simulink model "descriptor"  (R2015a)
settings: Solver=ode45  StartTime=0.0  StopTime=10.0  RelTol=1e-3
InitFcn:
  | %% DSPBuilder Start
  | alt_dspbuilder_update_model(bdroot)
  | %% DSPBuilder End
libraries: allblocks_alteradspbuilder2 x126
settings Model: Creator=ASUS  LastModifiedBy=ASUS

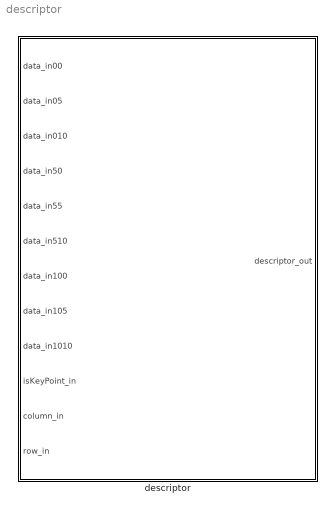
== system descriptor ==
  descriptor : Subsystem

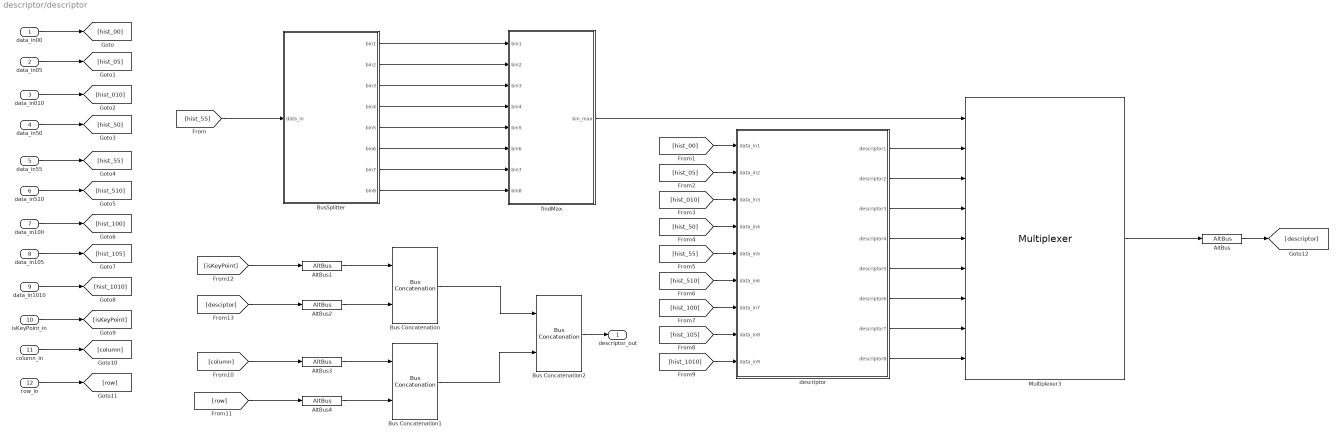
== system descriptor/descriptor ==
  data_in00 : Inport
  data_in05 : Inport  Port=2
  data_in010 : Inport  Port=3
  data_in50 : Inport  Port=4
  data_in55 : Inport  Port=5
  data_in510 : Inport  Port=6
  data_in100 : Inport  Port=7
  data_in105 : Inport  Port=8
  data_in1010 : Inport  Port=9
  isKeyPoint_in : Inport  Port=10
  column_in : Inport  Port=11
  row_in : Inport  Port=12
  AltBus : allblocks_alteradspbuilder2/AltBus  BusType=Unsigned Integer  bwl=128*9  bwr=0  saturate=off  floatingPointInput=on  floatingPointOutput=on  logOutputs=off  logFile=C:\Users\ASUS\Desktop\sift_fpga_final\Octave_1\tb_descriptor\descriptor_descriptor_AltBus.fixedpointlog
  AltBus1 : allblocks_alteradspbuilder2/AltBus  BusType=Single Bit  bwl=1  bwr=0  saturate=off  floatingPointInput=on  floatingPointOutput=on  logOutputs=off  logFile=C:\Users\ASUS\Desktop\sift_fpga_final\Octave_1\tb_descriptor\descriptor_descriptor_AltBus1.fixedpointlog
  AltBus2 : allblocks_alteradspbuilder2/AltBus  BusType=Unsigned Integer  bwl=128*9  bwr=0  saturate=off  floatingPointInput=on  floatingPointOutput=on  logOutputs=off  logFile=C:\Users\ASUS\Desktop\sift_fpga_final\Octave_1\tb_descriptor\descriptor_descriptor_AltBus2.fixedpointlog
  AltBus3 : allblocks_alteradspbuilder2/AltBus  BusType=Unsigned Integer  bwl=10  bwr=0  saturate=off  floatingPointInput=on  floatingPointOutput=on  logOutputs=off  logFile=C:\Users\ASUS\Desktop\sift_fpga_final\Octave_1\tb_descriptor\descriptor_descriptor_AltBus3.fixedpointlog
  AltBus4 : allblocks_alteradspbuilder2/AltBus  BusType=Unsigned Integer  bwl=10  bwr=0  saturate=off  floatingPointInput=on  floatingPointOutput=on  logOutputs=off  logFile=C:\Users\ASUS\Desktop\sift_fpga_final\Octave_1\tb_descriptor\descriptor_descriptor_AltBus4.fixedpointlog
  Bus Concatenation : allblocks_alteradspbuilder2/Bus Concatenation  isSigned=off  awidth=1  bwidth=128*9  pipeline_display=0
  Bus Concatenation1 : allblocks_alteradspbuilder2/Bus Concatenation  isSigned=off  awidth=10  bwidth=10  pipeline_display=0
  Bus Concatenation2 : allblocks_alteradspbuilder2/Bus Concatenation  isSigned=off  awidth=1153  bwidth=20  pipeline_display=0
  BusSplitter : Subsystem
  Multiplexer3 : allblocks_alteradspbuilder2/Multiplexer  numInputs=8  pipeline=0  oneHot=off  pipeline_display=0  use_ena=off  use_aclr=off  allowFloatingPointOverride=on  logOutputs=off  logFile=C:\Users\ASUS\Desktop\sift_fpga_final\Octave_1\tb_descriptor\descriptor_descriptor_Multiplexer3.fixedpointlog
  descriptor : Subsystem
  findMax : Subsystem
  descriptor_out : Outport
  wires:
  [hist_105] -> descriptor/8(data_in8)
  [hist_100] -> descriptor/7(data_in7)
  [hist_510] -> descriptor/6(data_in6)
  [hist_55] -> descriptor/5(data_in5)
  Multiplexer3/1 -> AltBus/1
  [hist_1010] -> descriptor/9(data_in9)
  descriptor/1(descriptor1) -> Multiplexer3/2
  [hist_05] -> descriptor/2(data_in2)
  [hist_010] -> descriptor/3(data_in3)
  [hist_50] -> descriptor/4(data_in4)
  descriptor/5(descriptor5) -> Multiplexer3/6
  descriptor/4(descriptor4) -> Multiplexer3/5
  [hist_00] -> descriptor/1(data_in1)
  descriptor/7(descriptor7) -> Multiplexer3/8
  descriptor/8(descriptor8) -> Multiplexer3/9
  descriptor/2(descriptor2) -> Multiplexer3/3
  descriptor/3(descriptor3) -> Multiplexer3/4
  descriptor/6(descriptor6) -> Multiplexer3/7
  BusSplitter/3(bin3) -> findMax/3(bin3)
  data_in00/1 -> [hist_00]
  data_in50/1 -> [hist_50]
  BusSplitter/1(bin1) -> findMax/1(bin1)
  data_in100/1 -> [hist_100]
  data_in010/1 -> [hist_010]
  data_in105/1 -> [hist_105]
  [hist_55] -> BusSplitter/1(data_in)
  data_in510/1 -> [hist_510]
  column_in/1 -> [column]
  data_in1010/1 -> [hist_1010]
  BusSplitter/8(bin8) -> findMax/8(bin8)
  findMax/1(bin_max) -> Multiplexer3/1
  data_in55/1 -> [hist_55]
  isKeyPoint_in/1 -> [isKeyPoint]
  row_in/1 -> [row]
  BusSplitter/4(bin4) -> findMax/4(bin4)
  BusSplitter/2(bin2) -> findMax/2(bin2)
  data_in05/1 -> [hist_05]
  BusSplitter/5(bin5) -> findMax/5(bin5)
  BusSplitter/7(bin7) -> findMax/7(bin7)
  BusSplitter/6(bin6) -> findMax/6(bin6)
  AltBus/1 -> [descriptor]
  [isKeyPoint] -> AltBus1/1
  [desciptor] -> AltBus2/1
  [column] -> AltBus3/1
  [row] -> AltBus4/1
  AltBus1/1 -> Bus Concatenation/1
  AltBus2/1 -> Bus Concatenation/2
  AltBus3/1 -> Bus Concatenation1/1
  AltBus4/1 -> Bus Concatenation1/2
  Bus Concatenation/1 -> Bus Concatenation2/1
  Bus Concatenation1/1 -> Bus Concatenation2/2
  Bus Concatenation2/1 -> descriptor_out/1

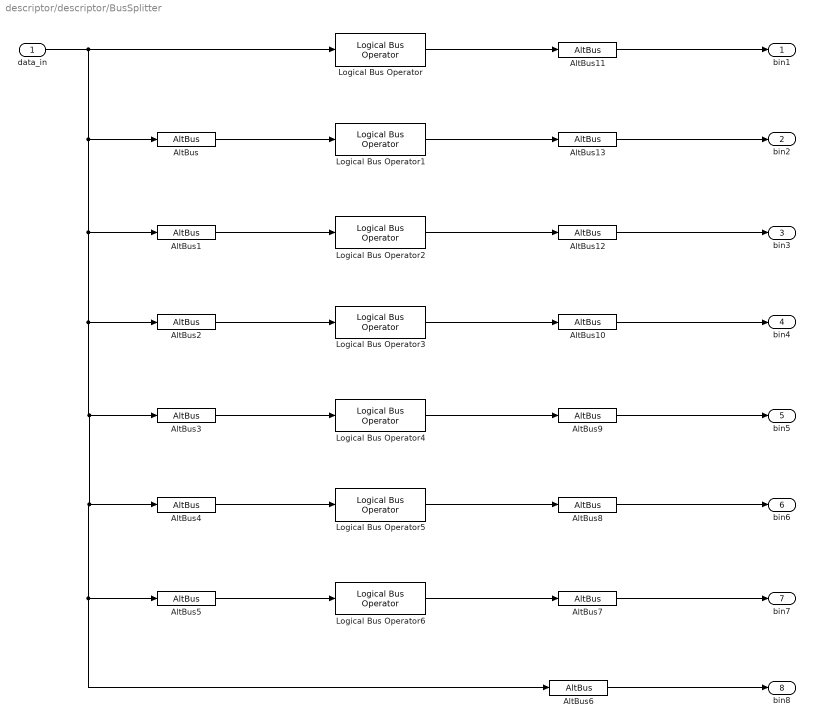
== system descriptor/descriptor/BusSplitter ==
  data_in : Inport
  AltBus : allblocks_alteradspbuilder2/AltBus  BusType=Unsigned Integer  bwl=112  bwr=0  saturate=off  floatingPointInput=on  floatingPointOutput=on  logOutputs=off  logFile=C:\Users\ASUS\Desktop\sift_fpga_final\Octave_1\tb_descriptor\descriptor_descriptor_BusSplitter_AltBus.fixedpointlog
  AltBus1 : allblocks_alteradspbuilder2/AltBus  BusType=Unsigned Integer  bwl=96  bwr=0  saturate=off  floatingPointInput=on  floatingPointOutput=on  logOutputs=off  logFile=C:\Users\ASUS\Desktop\sift_fpga_final\Octave_1\tb_descriptor\descriptor_descriptor_BusSplitter_AltBus1.fixedpointlog
  AltBus10 : allblocks_alteradspbuilder2/AltBus  BusType=Unsigned Integer  bwl=16  bwr=0  saturate=off  floatingPointInput=on  floatingPointOutput=on  logOutputs=off  logFile=C:\Users\ASUS\Desktop\sift_fpga_final\Octave_1\tb_descriptor\descriptor_descriptor_BusSplitter_AltBus10.fixedpointlog
  AltBus11 : allblocks_alteradspbuilder2/AltBus  BusType=Unsigned Integer  bwl=16  bwr=0  saturate=off  floatingPointInput=on  floatingPointOutput=on  logOutputs=off  logFile=C:\Users\ASUS\Desktop\sift_fpga_final\Octave_1\tb_descriptor\descriptor_descriptor_BusSplitter_AltBus11.fixedpointlog
  AltBus12 : allblocks_alteradspbuilder2/AltBus  BusType=Unsigned Integer  bwl=16  bwr=0  saturate=off  floatingPointInput=on  floatingPointOutput=on  logOutputs=off  logFile=C:\Users\ASUS\Desktop\sift_fpga_final\Octave_1\tb_descriptor\descriptor_descriptor_BusSplitter_AltBus12.fixedpointlog
  AltBus13 : allblocks_alteradspbuilder2/AltBus  BusType=Unsigned Integer  bwl=16  bwr=0  saturate=off  floatingPointInput=on  floatingPointOutput=on  logOutputs=off  logFile=C:\Users\ASUS\Desktop\sift_fpga_final\Octave_1\tb_descriptor\descriptor_descriptor_BusSplitter_AltBus13.fixedpointlog
  AltBus2 : allblocks_alteradspbuilder2/AltBus  BusType=Unsigned Integer  bwl=80  bwr=0  saturate=off  floatingPointInput=on  floatingPointOutput=on  logOutputs=off  logFile=C:\Users\ASUS\Desktop\sift_fpga_final\Octave_1\tb_descriptor\descriptor_descriptor_BusSplitter_AltBus2.fixedpointlog
  AltBus3 : allblocks_alteradspbuilder2/AltBus  BusType=Unsigned Integer  bwl=64  bwr=0  saturate=off  floatingPointInput=on  floatingPointOutput=on  logOutputs=off  logFile=C:\Users\ASUS\Desktop\sift_fpga_final\Octave_1\tb_descriptor\descriptor_descriptor_BusSplitter_AltBus3.fixedpointlog
  AltBus4 : allblocks_alteradspbuilder2/AltBus  BusType=Unsigned Integer  bwl=48  bwr=0  saturate=off  floatingPointInput=on  floatingPointOutput=on  logOutputs=off  logFile=C:\Users\ASUS\Desktop\sift_fpga_final\Octave_1\tb_descriptor\descriptor_descriptor_BusSplitter_AltBus4.fixedpointlog
  AltBus5 : allblocks_alteradspbuilder2/AltBus  BusType=Unsigned Integer  bwl=32  bwr=0  saturate=off  floatingPointInput=on  floatingPointOutput=on  logOutputs=off  logFile=C:\Users\ASUS\Desktop\sift_fpga_final\Octave_1\tb_descriptor\descriptor_descriptor_BusSplitter_AltBus5.fixedpointlog
  AltBus6 : allblocks_alteradspbuilder2/AltBus  BusType=Unsigned Integer  bwl=16  bwr=0  saturate=off  floatingPointInput=on  floatingPointOutput=on  logOutputs=off  logFile=C:\Users\ASUS\Desktop\sift_fpga_final\Octave_1\tb_descriptor\descriptor_descriptor_BusSplitter_AltBus6.fixedpointlog
  AltBus7 : allblocks_alteradspbuilder2/AltBus  BusType=Unsigned Integer  bwl=16  bwr=0  saturate=off  floatingPointInput=on  floatingPointOutput=on  logOutputs=off  logFile=C:\Users\ASUS\Desktop\sift_fpga_final\Octave_1\tb_descriptor\descriptor_descriptor_BusSplitter_AltBus7.fixedpointlog
  AltBus8 : allblocks_alteradspbuilder2/AltBus  BusType=Unsigned Integer  bwl=16  bwr=0  saturate=off  floatingPointInput=on  floatingPointOutput=on  logOutputs=off  logFile=C:\Users\ASUS\Desktop\sift_fpga_final\Octave_1\tb_descriptor\descriptor_descriptor_BusSplitter_AltBus8.fixedpointlog
  AltBus9 : allblocks_alteradspbuilder2/AltBus  BusType=Unsigned Integer  bwl=16  bwr=0  saturate=off  floatingPointInput=on  floatingPointOutput=on  logOutputs=off  logFile=C:\Users\ASUS\Desktop\sift_fpga_final\Octave_1\tb_descriptor\descriptor_descriptor_BusSplitter_AltBus9.fixedpointlog
  Logical Bus Operator : allblocks_alteradspbuilder2/Logical Bus Operator  BusType=Unsigned Integer  bwl=128  bwr=0  LogicalOp_text=Shift Right  mask_value_num=-5  shift_amount=112  force_sign_ext=on  pipeline_display=0
  Logical Bus Operator1 : allblocks_alteradspbuilder2/Logical Bus Operator  BusType=Unsigned Integer  bwl=112  bwr=0  LogicalOp_text=Shift Right  mask_value_num=-5  shift_amount=96  force_sign_ext=on  pipeline_display=0
  Logical Bus Operator2 : allblocks_alteradspbuilder2/Logical Bus Operator  BusType=Unsigned Integer  bwl=96  bwr=0  LogicalOp_text=Shift Right  mask_value_num=-5  shift_amount=80  force_sign_ext=on  pipeline_display=0
  Logical Bus Operator3 : allblocks_alteradspbuilder2/Logical Bus Operator  BusType=Unsigned Integer  bwl=80  bwr=0  LogicalOp_text=Shift Right  mask_value_num=-5  shift_amount=64  force_sign_ext=on  pipeline_display=0
  Logical Bus Operator4 : allblocks_alteradspbuilder2/Logical Bus Operator  BusType=Unsigned Integer  bwl=64  bwr=0  LogicalOp_text=Shift Right  mask_value_num=-5  shift_amount=48  force_sign_ext=on  pipeline_display=0
  Logical Bus Operator5 : allblocks_alteradspbuilder2/Logical Bus Operator  BusType=Unsigned Integer  bwl=48  bwr=0  LogicalOp_text=Shift Right  mask_value_num=-5  shift_amount=32  force_sign_ext=on  pipeline_display=0
  Logical Bus Operator6 : allblocks_alteradspbuilder2/Logical Bus Operator  BusType=Unsigned Integer  bwl=32  bwr=0  LogicalOp_text=Shift Right  mask_value_num=-5  shift_amount=16  force_sign_ext=on  pipeline_display=0
  bin1 : Outport
  bin2 : Outport  Port=2
  bin3 : Outport  Port=3
  bin4 : Outport  Port=4
  bin5 : Outport  Port=5
  bin6 : Outport  Port=6
  bin7 : Outport  Port=7
  bin8 : Outport  Port=8
  wires:
  Logical Bus Operator6/1 -> AltBus7/1
  AltBus1/1 -> Logical Bus Operator2/1
  AltBus9/1 -> bin5/1
  AltBus8/1 -> bin6/1
  AltBus7/1 -> bin7/1
  AltBus6/1 -> bin8/1
  AltBus13/1 -> bin2/1
  AltBus/1 -> Logical Bus Operator1/1
  AltBus10/1 -> bin4/1
  AltBus12/1 -> bin3/1
  AltBus11/1 -> bin1/1
  AltBus3/1 -> Logical Bus Operator4/1
  AltBus2/1 -> Logical Bus Operator3/1
  AltBus4/1 -> Logical Bus Operator5/1
  data_in/1 -> AltBus6/1, AltBus5/1, AltBus4/1, AltBus3/1, AltBus2/1, AltBus1/1, AltBus/1, Logical Bus Operator/1
  AltBus5/1 -> Logical Bus Operator6/1
  Logical Bus Operator1/1 -> AltBus13/1
  Logical Bus Operator2/1 -> AltBus12/1
  Logical Bus Operator/1 -> AltBus11/1
  Logical Bus Operator5/1 -> AltBus8/1
  Logical Bus Operator4/1 -> AltBus9/1
  Logical Bus Operator3/1 -> AltBus10/1

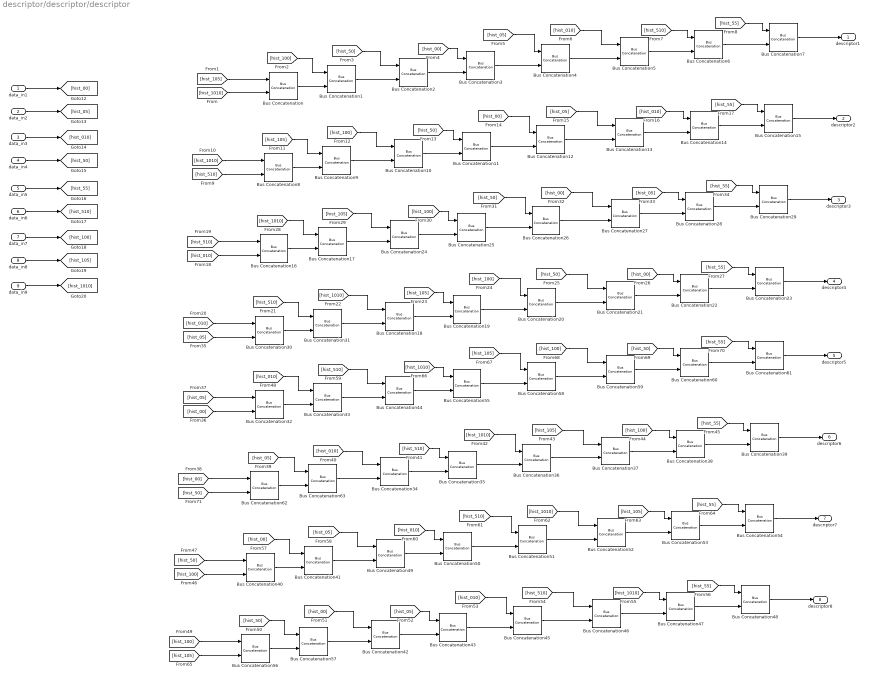
== system descriptor/descriptor/descriptor ==
  data_in1 : Inport
  data_in2 : Inport  Port=2
  data_in3 : Inport  Port=3
  data_in4 : Inport  Port=4
  data_in5 : Inport  Port=5
  data_in6 : Inport  Port=6
  data_in7 : Inport  Port=7
  data_in8 : Inport  Port=8
  data_in9 : Inport  Port=9
  Bus Concatenation{,8,16,30,32,40,56,62} (8 alike) : allblocks_alteradspbuilder2/Bus Concatenation  isSigned=off  awidth=128  bwidth=128  pipeline_display=0
  Bus Concatenation{1,9,17,31,33,41,57,63} (8 alike) : allblocks_alteradspbuilder2/Bus Concatenation  isSigned=off  awidth=128  bwidth=256  pipeline_display=0
  Bus Concatenation{2,10,18,24,34,42,44,49} (8 alike) : allblocks_alteradspbuilder2/Bus Concatenation  isSigned=off  awidth=128  bwidth=384  pipeline_display=0
  Bus Concatenation{3,11,19,25,35,43,50,55} (8 alike) : allblocks_alteradspbuilder2/Bus Concatenation  isSigned=off  awidth=128  bwidth=512  pipeline_display=0
  Bus Concatenation{4,12,20,26,36,45,51,58} (8 alike) : allblocks_alteradspbuilder2/Bus Concatenation  isSigned=off  awidth=128  bwidth=640  pipeline_display=0
  Bus Concatenation{5,13,21,27,37,46,52,59} (8 alike) : allblocks_alteradspbuilder2/Bus Concatenation  isSigned=off  awidth=128  bwidth=768  pipeline_display=0
  Bus Concatenation{6,14,22,28,38,47,53,60} (8 alike) : allblocks_alteradspbuilder2/Bus Concatenation  isSigned=off  awidth=128  bwidth=896  pipeline_display=0
  Bus Concatenation{7,15,23,29,39,48,54,61} (8 alike) : allblocks_alteradspbuilder2/Bus Concatenation  isSigned=off  awidth=128  bwidth=1024  pipeline_display=0
  descriptor1 : Outport
  descriptor2 : Outport  Port=2
  descriptor3 : Outport  Port=3
  descriptor4 : Outport  Port=4
  descriptor5 : Outport  Port=5
  descriptor6 : Outport  Port=6
  descriptor7 : Outport  Port=7
  descriptor8 : Outport  Port=8
  wires:
  data_in2/1 -> [hist_05]
  data_in4/1 -> [hist_50]
  data_in6/1 -> [hist_510]
  data_in5/1 -> [hist_55]
  data_in7/1 -> [hist_100]
  data_in8/1 -> [hist_105]
  data_in3/1 -> [hist_010]
  data_in1/1 -> [hist_00]
  data_in9/1 -> [hist_1010]
  Bus Concatenation3/1 -> Bus Concatenation4/2
  Bus Concatenation4/1 -> Bus Concatenation5/2
  Bus Concatenation5/1 -> Bus Concatenation6/2
  Bus Concatenation/1 -> Bus Concatenation1/2
  [hist_100] -> Bus Concatenation1/1
  Bus Concatenation1/1 -> Bus Concatenation2/2
  [hist_1010] -> Bus Concatenation/2
  [hist_50] -> Bus Concatenation2/1
  [hist_105] -> Bus Concatenation/1
  Bus Concatenation2/1 -> Bus Concatenation3/2
  [hist_00] -> Bus Concatenation3/1
  [hist_05] -> Bus Concatenation4/1
  [hist_010] -> Bus Concatenation5/1
  [hist_510] -> Bus Concatenation6/1
  Bus Concatenation6/1 -> Bus Concatenation7/2
  [hist_55] -> Bus Concatenation7/1
  Bus Concatenation7/1 -> descriptor1/1
  Bus Concatenation11/1 -> Bus Concatenation12/2
  Bus Concatenation12/1 -> Bus Concatenation13/2
  Bus Concatenation13/1 -> Bus Concatenation14/2
  Bus Concatenation8/1 -> Bus Concatenation9/2
  [hist_105] -> Bus Concatenation9/1
  Bus Concatenation9/1 -> Bus Concatenation10/2
  [hist_510] -> Bus Concatenation8/2
  [hist_100] -> Bus Concatenation10/1
  [hist_1010] -> Bus Concatenation8/1
  Bus Concatenation10/1 -> Bus Concatenation11/2
  [hist_50] -> Bus Concatenation11/1
  [hist_00] -> Bus Concatenation12/1
  [hist_05] -> Bus Concatenation13/1
  [hist_010] -> Bus Concatenation14/1
  Bus Concatenation14/1 -> Bus Concatenation15/2
  [hist_55] -> Bus Concatenation15/1
  Bus Concatenation15/1 -> descriptor2/1
  Bus Concatenation25/1 -> Bus Concatenation26/2
  Bus Concatenation26/1 -> Bus Concatenation27/2
  Bus Concatenation27/1 -> Bus Concatenation28/2
  Bus Concatenation16/1 -> Bus Concatenation17/2
  [hist_1010] -> Bus Concatenation17/1
  Bus Concatenation17/1 -> Bus Concatenation24/2
  [hist_010] -> Bus Concatenation16/2
  [hist_105] -> Bus Concatenation24/1
  [hist_510] -> Bus Concatenation16/1
  Bus Concatenation24/1 -> Bus Concatenation25/2
  [hist_100] -> Bus Concatenation25/1
  [hist_50] -> Bus Concatenation26/1
  [hist_00] -> Bus Concatenation27/1
  [hist_05] -> Bus Concatenation28/1
  Bus Concatenation28/1 -> Bus Concatenation29/2
  [hist_55] -> Bus Concatenation29/1
  Bus Concatenation29/1 -> descriptor3/1
  Bus Concatenation19/1 -> Bus Concatenation20/2
  Bus Concatenation20/1 -> Bus Concatenation21/2
  Bus Concatenation21/1 -> Bus Concatenation22/2
  Bus Concatenation30/1 -> Bus Concatenation31/2
  [hist_510] -> Bus Concatenation31/1
  Bus Concatenation31/1 -> Bus Concatenation18/2
  [hist_05] -> Bus Concatenation30/2
  [hist_1010] -> Bus Concatenation18/1
  [hist_010] -> Bus Concatenation30/1
  Bus Concatenation18/1 -> Bus Concatenation19/2
  [hist_105] -> Bus Concatenation19/1
  [hist_100] -> Bus Concatenation20/1
  [hist_50] -> Bus Concatenation21/1
  [hist_00] -> Bus Concatenation22/1
  Bus Concatenation22/1 -> Bus Concatenation23/2
  [hist_55] -> Bus Concatenation23/1
  Bus Concatenation23/1 -> descriptor4/1
  Bus Concatenation55/1 -> Bus Concatenation58/2
  Bus Concatenation58/1 -> Bus Concatenation59/2
  Bus Concatenation59/1 -> Bus Concatenation60/2
  Bus Concatenation32/1 -> Bus Concatenation33/2
  [hist_010] -> Bus Concatenation33/1
  Bus Concatenation33/1 -> Bus Concatenation44/2
  [hist_00] -> Bus Concatenation32/2
  [hist_510] -> Bus Concatenation44/1
  [hist_05] -> Bus Concatenation32/1
  Bus Concatenation44/1 -> Bus Concatenation55/2
  [hist_1010] -> Bus Concatenation55/1
  [hist_105] -> Bus Concatenation58/1
  [hist_100] -> Bus Concatenation59/1
  [hist_50] -> Bus Concatenation60/1
  Bus Concatenation60/1 -> Bus Concatenation61/2
  [hist_55] -> Bus Concatenation61/1
  Bus Concatenation61/1 -> descriptor5/1
  Bus Concatenation35/1 -> Bus Concatenation36/2
  Bus Concatenation36/1 -> Bus Concatenation37/2
  Bus Concatenation37/1 -> Bus Concatenation38/2
  Bus Concatenation62/1 -> Bus Concatenation63/2
  [hist_05] -> Bus Concatenation63/1
  Bus Concatenation63/1 -> Bus Concatenation34/2
  [hist_50] -> Bus Concatenation62/2
  [hist_010] -> Bus Concatenation34/1
  [hist_00] -> Bus Concatenation62/1
  Bus Concatenation34/1 -> Bus Concatenation35/2
  [hist_510] -> Bus Concatenation35/1
  [hist_1010] -> Bus Concatenation36/1
  [hist_105] -> Bus Concatenation37/1
  [hist_100] -> Bus Concatenation38/1
  Bus Concatenation38/1 -> Bus Concatenation39/2
  [hist_55] -> Bus Concatenation39/1
  Bus Concatenation39/1 -> descriptor6/1
  Bus Concatenation50/1 -> Bus Concatenation51/2
  Bus Concatenation51/1 -> Bus Concatenation52/2
  Bus Concatenation52/1 -> Bus Concatenation53/2
  Bus Concatenation40/1 -> Bus Concatenation41/2
  [hist_00] -> Bus Concatenation41/1
  Bus Concatenation41/1 -> Bus Concatenation49/2
  [hist_100] -> Bus Concatenation40/2
  [hist_05] -> Bus Concatenation49/1
  [hist_50] -> Bus Concatenation40/1
  Bus Concatenation49/1 -> Bus Concatenation50/2
  [hist_010] -> Bus Concatenation50/1
  [hist_510] -> Bus Concatenation51/1
  [hist_1010] -> Bus Concatenation52/1
  [hist_105] -> Bus Concatenation53/1
  Bus Concatenation53/1 -> Bus Concatenation54/2
  [hist_55] -> Bus Concatenation54/1
  Bus Concatenation54/1 -> descriptor7/1
  Bus Concatenation43/1 -> Bus Concatenation45/2
  Bus Concatenation45/1 -> Bus Concatenation46/2
  Bus Concatenation46/1 -> Bus Concatenation47/2
  Bus Concatenation56/1 -> Bus Concatenation57/2
  [hist_50] -> Bus Concatenation57/1
  Bus Concatenation57/1 -> Bus Concatenation42/2
  [hist_105] -> Bus Concatenation56/2
  [hist_00] -> Bus Concatenation42/1
  [hist_100] -> Bus Concatenation56/1
  Bus Concatenation42/1 -> Bus Concatenation43/2
  [hist_05] -> Bus Concatenation43/1
  [hist_010] -> Bus Concatenation45/1
  [hist_510] -> Bus Concatenation46/1
  [hist_1010] -> Bus Concatenation47/1
  Bus Concatenation47/1 -> Bus Concatenation48/2
  [hist_55] -> Bus Concatenation48/1
  Bus Concatenation48/1 -> descriptor8/1

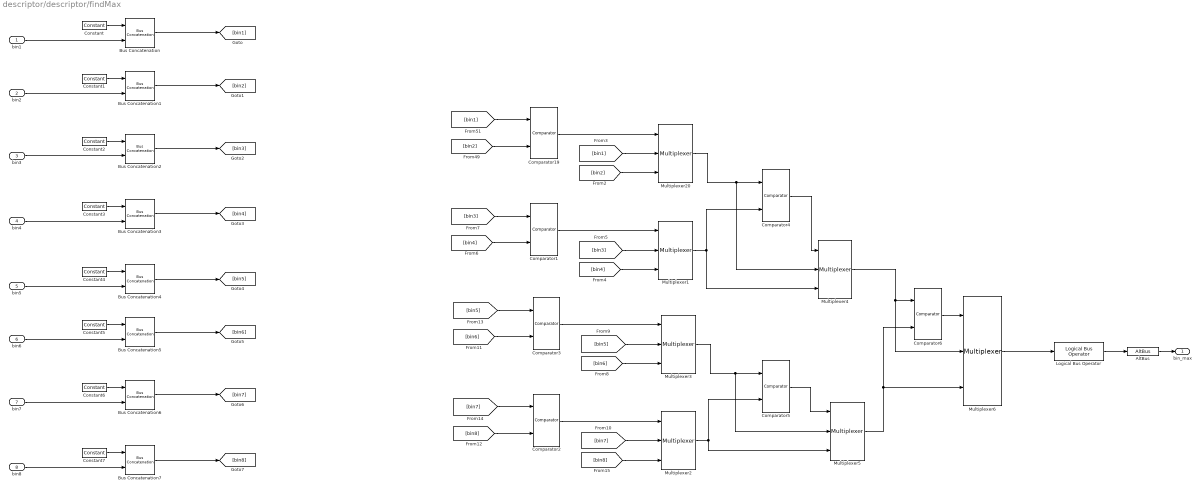
== system descriptor/descriptor/findMax ==
  bin1 : Inport
  bin2 : Inport  Port=2
  bin3 : Inport  Port=3
  bin4 : Inport  Port=4
  bin5 : Inport  Port=5
  bin6 : Inport  Port=6
  bin7 : Inport  Port=7
  bin8 : Inport  Port=8
  AltBus : allblocks_alteradspbuilder2/AltBus  BusType=Unsigned Integer  bwl=3  bwr=0  saturate=off  floatingPointInput=on  floatingPointOutput=on  logOutputs=off  logFile=C:\Users\ASUS\Desktop\sift_fpga_final\Octave_1\tb_descriptor\descriptor_descriptor_findMax_AltBus.fixedpointlog
  Bus Concatenation{,1..7} (8 alike) : allblocks_alteradspbuilder2/Bus Concatenation  isSigned=off  awidth=3  bwidth=16  pipeline_display=0
  Comparator1 : allblocks_alteradspbuilder2/Comparator  direction=a < b  pipeline_display=0  allowFloatingPointOverride=on  logOutputs=off  logFile=C:\Users\ASUS\Desktop\sift_fpga_final\Octave_1\tb_descriptor\descriptor_descriptor_findMax_Comparator1.fixedpointlog
  Comparator19 : allblocks_alteradspbuilder2/Comparator  direction=a < b  pipeline_display=0  allowFloatingPointOverride=on  logOutputs=off  logFile=C:\Users\ASUS\Desktop\sift_fpga_final\Octave_1\tb_descriptor\descriptor_descriptor_findMax_Comparator19.fixedpointlog
  Comparator2 : allblocks_alteradspbuilder2/Comparator  direction=a < b  pipeline_display=0  allowFloatingPointOverride=on  logOutputs=off  logFile=C:\Users\ASUS\Desktop\sift_fpga_final\Octave_1\tb_descriptor\descriptor_descriptor_findMax_Comparator2.fixedpointlog
  Comparator3 : allblocks_alteradspbuilder2/Comparator  direction=a < b  pipeline_display=0  allowFloatingPointOverride=on  logOutputs=off  logFile=C:\Users\ASUS\Desktop\sift_fpga_final\Octave_1\tb_descriptor\descriptor_descriptor_findMax_Comparator3.fixedpointlog
  Comparator4 : allblocks_alteradspbuilder2/Comparator  direction=a < b  pipeline_display=0  allowFloatingPointOverride=on  logOutputs=off  logFile=C:\Users\ASUS\Desktop\sift_fpga_final\Octave_1\tb_descriptor\descriptor_descriptor_findMax_Comparator4.fixedpointlog
  Comparator5 : allblocks_alteradspbuilder2/Comparator  direction=a < b  pipeline_display=0  allowFloatingPointOverride=on  logOutputs=off  logFile=C:\Users\ASUS\Desktop\sift_fpga_final\Octave_1\tb_descriptor\descriptor_descriptor_findMax_Comparator5.fixedpointlog
  Comparator6 : allblocks_alteradspbuilder2/Comparator  direction=a < b  pipeline_display=0  allowFloatingPointOverride=on  logOutputs=off  logFile=C:\Users\ASUS\Desktop\sift_fpga_final\Octave_1\tb_descriptor\descriptor_descriptor_findMax_Comparator6.fixedpointlog
  Constant : allblocks_alteradspbuilder2/Constant  mask_cst=0  BusType=Unsigned Integer  bwl=3  bwr=0  roundMode=Truncate  satMode=Wrap  SpecifyClock=off  allowFloatingPointOverride=on  logOutputs=off  logFile=C:\Users\ASUS\Desktop\sift_fpga_final\Octave_1\tb_descriptor\descriptor_descriptor_findMax_Constant.fixedpointlog
  Constant1 : allblocks_alteradspbuilder2/Constant  mask_cst=1  BusType=Unsigned Integer  bwl=3  bwr=0  roundMode=Truncate  satMode=Wrap  SpecifyClock=off  allowFloatingPointOverride=on  logOutputs=off  logFile=C:\Users\ASUS\Desktop\sift_fpga_final\Octave_1\tb_descriptor\descriptor_descriptor_findMax_Constant1.fixedpointlog
  Constant2 : allblocks_alteradspbuilder2/Constant  mask_cst=2  BusType=Unsigned Integer  bwl=3  bwr=0  roundMode=Truncate  satMode=Wrap  SpecifyClock=off  allowFloatingPointOverride=on  logOutputs=off  logFile=C:\Users\ASUS\Desktop\sift_fpga_final\Octave_1\tb_descriptor\descriptor_descriptor_findMax_Constant2.fixedpointlog
  Constant3 : allblocks_alteradspbuilder2/Constant  mask_cst=3  BusType=Unsigned Integer  bwl=3  bwr=0  roundMode=Truncate  satMode=Wrap  SpecifyClock=off  allowFloatingPointOverride=on  logOutputs=off  logFile=C:\Users\ASUS\Desktop\sift_fpga_final\Octave_1\tb_descriptor\descriptor_descriptor_findMax_Constant3.fixedpointlog
  Constant4 : allblocks_alteradspbuilder2/Constant  mask_cst=4  BusType=Unsigned Integer  bwl=3  bwr=0  roundMode=Truncate  satMode=Wrap  SpecifyClock=off  allowFloatingPointOverride=on  logOutputs=off  logFile=C:\Users\ASUS\Desktop\sift_fpga_final\Octave_1\tb_descriptor\descriptor_descriptor_findMax_Constant4.fixedpointlog
  Constant5 : allblocks_alteradspbuilder2/Constant  mask_cst=5  BusType=Unsigned Integer  bwl=3  bwr=0  roundMode=Truncate  satMode=Wrap  SpecifyClock=off  allowFloatingPointOverride=on  logOutputs=off  logFile=C:\Users\ASUS\Desktop\sift_fpga_final\Octave_1\tb_descriptor\descriptor_descriptor_findMax_Constant5.fixedpointlog
  Constant6 : allblocks_alteradspbuilder2/Constant  mask_cst=6  BusType=Unsigned Integer  bwl=3  bwr=0  roundMode=Truncate  satMode=Wrap  SpecifyClock=off  allowFloatingPointOverride=on  logOutputs=off  logFile=C:\Users\ASUS\Desktop\sift_fpga_final\Octave_1\tb_descriptor\descriptor_descriptor_findMax_Constant6.fixedpointlog
  Constant7 : allblocks_alteradspbuilder2/Constant  mask_cst=7  BusType=Unsigned Integer  bwl=3  bwr=0  roundMode=Truncate  satMode=Wrap  SpecifyClock=off  allowFloatingPointOverride=on  logOutputs=off  logFile=C:\Users\ASUS\Desktop\sift_fpga_final\Octave_1\tb_descriptor\descriptor_descriptor_findMax_Constant7.fixedpointlog
  Logical Bus Operator : allblocks_alteradspbuilder2/Logical Bus Operator  BusType=Unsigned Integer  bwl=19  bwr=0  LogicalOp_text=Shift Right  mask_value_num=-5  shift_amount=16  force_sign_ext=on  pipeline_display=0
  Multiplexer1 : allblocks_alteradspbuilder2/Multiplexer  numInputs=2  pipeline=0  oneHot=off  pipeline_display=0  use_ena=off  use_aclr=off  allowFloatingPointOverride=on  logOutputs=off  logFile=C:\Users\ASUS\Desktop\sift_fpga_final\Octave_1\tb_descriptor\descriptor_descriptor_findMax_Multiplexer1.fixedpointlog
  Multiplexer2 : allblocks_alteradspbuilder2/Multiplexer  numInputs=2  pipeline=0  oneHot=off  pipeline_display=0  use_ena=off  use_aclr=off  allowFloatingPointOverride=on  logOutputs=off  logFile=C:\Users\ASUS\Desktop\sift_fpga_final\Octave_1\tb_descriptor\descriptor_descriptor_findMax_Multiplexer2.fixedpointlog
  Multiplexer20 : allblocks_alteradspbuilder2/Multiplexer  numInputs=2  pipeline=0  oneHot=off  pipeline_display=0  use_ena=off  use_aclr=off  allowFloatingPointOverride=on  logOutputs=off  logFile=C:\Users\ASUS\Desktop\sift_fpga_final\Octave_1\tb_descriptor\descriptor_descriptor_findMax_Multiplexer20.fixedpointlog
  Multiplexer3 : allblocks_alteradspbuilder2/Multiplexer  numInputs=2  pipeline=0  oneHot=off  pipeline_display=0  use_ena=off  use_aclr=off  allowFloatingPointOverride=on  logOutputs=off  logFile=C:\Users\ASUS\Desktop\sift_fpga_final\Octave_1\tb_descriptor\descriptor_descriptor_findMax_Multiplexer3.fixedpointlog
  Multiplexer4 : allblocks_alteradspbuilder2/Multiplexer  numInputs=2  pipeline=0  oneHot=off  pipeline_display=0  use_ena=off  use_aclr=off  allowFloatingPointOverride=on  logOutputs=off  logFile=C:\Users\ASUS\Desktop\sift_fpga_final\Octave_1\tb_descriptor\descriptor_descriptor_findMax_Multiplexer4.fixedpointlog
  Multiplexer5 : allblocks_alteradspbuilder2/Multiplexer  numInputs=2  pipeline=0  oneHot=off  pipeline_display=0  use_ena=off  use_aclr=off  allowFloatingPointOverride=on  logOutputs=off  logFile=C:\Users\ASUS\Desktop\sift_fpga_final\Octave_1\tb_descriptor\descriptor_descriptor_findMax_Multiplexer5.fixedpointlog
  Multiplexer6 : allblocks_alteradspbuilder2/Multiplexer  numInputs=2  pipeline=0  oneHot=off  pipeline_display=0  use_ena=off  use_aclr=off  allowFloatingPointOverride=on  logOutputs=off  logFile=C:\Users\ASUS\Desktop\sift_fpga_final\Octave_1\tb_descriptor\descriptor_descriptor_findMax_Multiplexer6.fixedpointlog
  bin_max : Outport
  wires:
  [bin1] -> Comparator19/1
  [bin2] -> Comparator19/2
  Comparator19/1 -> Multiplexer20/1
  [bin1] -> Multiplexer20/2
  [bin2] -> Multiplexer20/3
  Multiplexer20/1 -> Comparator4/1, Multiplexer4/2
  [bin3] -> Comparator1/1
  [bin4] -> Comparator1/2
  Comparator1/1 -> Multiplexer1/1
  [bin3] -> Multiplexer1/2
  [bin4] -> Multiplexer1/3
  Multiplexer1/1 -> Multiplexer4/3, Comparator4/2
  [bin5] -> Comparator3/1
  [bin6] -> Comparator3/2
  Comparator3/1 -> Multiplexer3/1
  [bin5] -> Multiplexer3/2
  [bin6] -> Multiplexer3/3
  Multiplexer3/1 -> Comparator5/1, Multiplexer5/2
  [bin7] -> Comparator2/1
  [bin8] -> Comparator2/2
  Comparator2/1 -> Multiplexer2/1
  [bin7] -> Multiplexer2/2
  [bin8] -> Multiplexer2/3
  Multiplexer2/1 -> Multiplexer5/3, Comparator5/2
  Comparator4/1 -> Multiplexer4/1
  Comparator5/1 -> Multiplexer5/1
  Multiplexer4/1 -> Multiplexer6/2, Comparator6/1
  Multiplexer5/1 -> Comparator6/2, Multiplexer6/3
  Comparator6/1 -> Multiplexer6/1
  bin1/1 -> Bus Concatenation/2
  Constant/1 -> Bus Concatenation/1
  Bus Concatenation/1 -> [bin1]
  bin2/1 -> Bus Concatenation1/2
  Constant1/1 -> Bus Concatenation1/1
  Bus Concatenation1/1 -> [bin2]
  bin3/1 -> Bus Concatenation2/2
  Constant2/1 -> Bus Concatenation2/1
  Bus Concatenation2/1 -> [bin3]
  bin4/1 -> Bus Concatenation3/2
  Constant3/1 -> Bus Concatenation3/1
  Bus Concatenation3/1 -> [bin4]
  bin5/1 -> Bus Concatenation4/2
  Constant4/1 -> Bus Concatenation4/1
  Bus Concatenation4/1 -> [bin5]
  bin6/1 -> Bus Concatenation5/2
  Constant5/1 -> Bus Concatenation5/1
  Bus Concatenation5/1 -> [bin6]
  bin7/1 -> Bus Concatenation6/2
  Constant6/1 -> Bus Concatenation6/1
  Bus Concatenation6/1 -> [bin7]
  bin8/1 -> Bus Concatenation7/2
  Constant7/1 -> Bus Concatenation7/1
  Bus Concatenation7/1 -> [bin8]
  Multiplexer6/1 -> Logical Bus Operator/1
  Logical Bus Operator/1 -> AltBus/1
  AltBus/1 -> bin_max/1
